simulink model "lab_sim"  (R2016a)
settings: Solver=VariableStepAuto  StartTime=0.0  StopTime=10.0  RelTol=1e-3
values from neighbouring files (symbols this model uses):
  A = [0, 1, 0, 0 ... (first row only)    [lab.m]
  B = [0 ... (first row only)    [lab.m]
  C = [1, 0, 0, 0 ... (first row only)    [lab.m]
  F = -acker(A, B, eign_F)    [lab.m]
  Init_cond = [0.1; 0; 0.1; 0]    [lab.m]
settings Model: Creator=gkbb  LastModifiedBy=gkbb

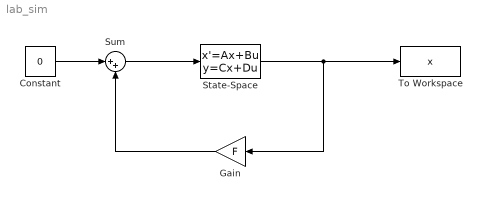
== system lab_sim ==
  Constant : Constant  Value=0
  Gain : Gain  Gain=F
  State-Space : StateSpace  A=A  B=B  C=C  D=0  X0=Init_cond
  Sum : Sum  Inputs=|++
  To Workspace : ToWorkspace  VariableName=x  SaveFormat=Timeseries  SampleTime=-1
  wires:
  Constant/1 -> Sum/1
  Sum/1 -> State-Space/1
  State-Space/1 -> Gain/1, To Workspace/1
  Gain/1 -> Sum/2
